simulink model "CurrentComp_LR_Vshunt_fb_v60"  (R2013a)
settings: Solver=ode23  StartTime=0.0  StopTime=1.2e-4  FixedStep=FS/50  MaxStep=1e-6  RelTol=1e-3  AbsTol=1e-5
InitFcn:
  | param=evalin('base','param;');
  | 
  | JR=str2num(param.JR);
  | KMT=str2num(param.KMT);
  | Rc=str2num(param.Rc);
  | Lc=str2num(param.Lc);
  | KFR=str2num(param.KFR);
  | KTB=str2num(param.KTB);
  | KBM=str2num(param.KBM);
  | Rsh=str2num(param.Rsh);
StartFcn:
  | sprintf('Info (%s):\nKTB = %.1e\nKBM = %.1e\n', gcs, KTB, KBM)
model workspace (MATLAB code in the model file):
  | %param=evalin('base','loadGalvoParam(4);');
  | param=evalin('base','param;');
  | 
  | JR=str2num(param.JR);
  | KMT=str2num(param.KMT);
  | Rc=str2num(param.Rc);
  | Lc=str2num(param.Lc);
  | KFR=str2num(param.KFR);
  | KTB=str2num(param.KTB);
  | KBM=str2num(param.KBM);
  | Rsh=str2num(param.Rsh);
libraries: simulink x1
settings Model: BufferReuse=off  Creator=mainster  LastModifiedBy=mainster
settings DataIOCC: SaveOutput=off  SaveTime=off
settings OptimizationCC: BlockReduction=off  InlineParams=on  OptimizeBlockIOStorage=off  BufferReuse=off  ExpressionFolding=off  LocalBlockOutputs=off
settings DebuggingCC: InitInArrayFormatMsg=none
settings ModelReferenceCC: ModelReferenceNumInstancesAllowed=Single  ModelReferenceMinAlgLoopOccurrences=on

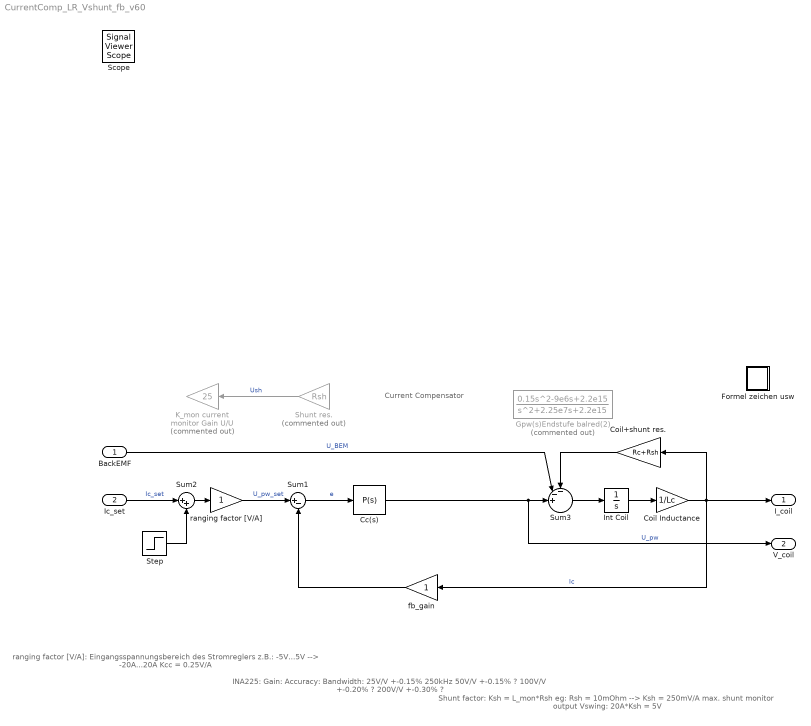
== system CurrentComp_LR_Vshunt_fb_v60 ==
  note: ranging factor [V/A]:
      | Eingangsspannungsbereich des
      | Stromreglers z.B.:
      | -5V...5V --> -20A...20A
      | Kcc = 0.25V/A
  note: Shunt factor:
      | Ksh = L_mon*Rsh
      |
      | eg: Rsh = 10mOhm
      |
      | --> Ksh = 250mV/A
      | max. shunt monitor
      | output Vswing:
      | 20A*Ksh = 5V
  note: INA225:
      | Gain:		Accuracy:		Bandwidth:
      | 25V/V		+-0.15%		250kHz
      | 50V/V		+-0.15%		?
      | 100V/V	+-0.20%		?
      | 200V/V	+-0.30%		?
  note: Current Compensator
  BackEMF : Inport
  Ic_set : Inport  Port=2
  Cc(s) : simulink/Continuous/PID Controller  Controller=P  TimeDomain=Continuous-time  SampleTime=-1  IntegratorMethod=Forward Euler  FilterMethod=Forward Euler  Form=Ideal  P=37.1538329650542  I=1985.39023021624  D=0  N=100  InitialConditionSource=internal  InitialConditionForIntegrator=0  InitialConditionForFilter=0  ExternalReset=none  LimitOutput=off  UpperSaturationLimit=inf  LowerSaturationLimit=-inf  LinearizeAsGain=on  AntiWindupMode=none  Kb=1  TrackingMode=off  Kt=1  PParamMin=[]  PParamMax=[]  IParamMin=[]  IParamMax=[]  DParamMin=[]  DParamMax=[]  NParamMin=[]  NParamMax=[]  KbParamMin=[]  KbParamMax=[]  KtParamMin=[]  KtParamMax=[]  POutMin=[]  POutMax=[]  IOutMin=[]  IOutMax=[]  DOutMin=[]  DOutMax=[]  NOutMin=[]  NOutMax=[]  KbOutMin=[]  KbOutMax=[]  KtOutMin=[]  KtOutMax=[]  IntegratorOutMin=[]  IntegratorOutMax=[]  FilterOutMin=[]  FilterOutMax=[]  SumOutMin=[]  SumOutMax=[]  SumI1OutMin=[]  SumI1OutMax=[]  SumI2OutMin=[]  SumI2OutMax=[]  SumI3OutMin=[]  SumI3OutMax=[]  SumDOutMin=[]  SumDOutMax=[]  SaturationOutMin=[]  SaturationOutMax=[]  IntegratorContinuousStateAttributes=''  IntegratorStateMustResolveToSignalObject=off  IntegratorRTWStateStorageClass=Auto  FilterContinuousStateAttributes=''  FilterStateMustResolveToSignalObject=off  FilterRTWStateStorageClass=Auto
      settings: AttributesFormatString=P = %<P>
  Coil Inductance : Gain  Gain=1/Lc
  Coil+shunt res. : Gain  Gain=Rc+Rsh
  Formel zeichen usw : Subsystem
  Gpw(s)Endstufe balred(2) : TransferFcn  Commented=on  Numerator=[0.15 -9e6 2.2e15]  Denominator=[1 2.25e7 2.2e15]
  Int Coil : Integrator
  K_mon current monitor Gain U/U : Gain  Commented=on  Gain=25
  Shunt res. : Gain  Commented=on  Gain=Rsh
  Step : Step  Time=0
      settings: AttributesFormatString=%<Time>
  Sum1 : Sum  Inputs=|+-
  Sum2 : Sum  Inputs=|++
  Sum3 : Sum  Inputs=--+||
  fb_gain : Gain
  ranging factor [V/A] : Gain
  I_coil : Outport
  V_coil : Outport  Port=2
  Scope : SignalViewerScope  IOType=viewer  RefreshTime=0.035000
      settings: ShowLegends=on  TimeRange=0.00014  YMin=-0.1  YMax=0.3
  wires:
  Ic_set/1 -> Sum2/1  "Ic_set"
  Sum1/1 -> Cc(s)/1  "e"
  Coil Inductance/1 -> fb_gain/1, I_coil/1, Coil+shunt res./1  "Ic"
  Sum3/1 -> Int Coil/1
  Int Coil/1 -> Coil Inductance/1
  Cc(s)/1 -> V_coil/1, Sum3/3  "U_pw"
  fb_gain/1 -> Sum1/2
  BackEMF/1 -> Sum3/2  "U_BEM"
  Coil+shunt res./1 -> Sum3/1
  ranging factor [V/A]/1 -> Sum1/1  "U_pw_set"
  Sum2/1 -> ranging factor [V/A]/1
  Step/1 -> Sum2/2
  Shunt res./1 -> K_mon current monitor Gain U/U/1  "Ush"

== system CurrentComp_LR_Vshunt_fb_v60/Formel zeichen usw ==
  note: Te: 		electrical torque, gen. by coils		[Nm]
      |  Ic: 			coil current							[A]
      |  Tfr:		rotor dynamic friction torque 		[Nm]
      |  Trb:		torsion bar torque					[Nm]
      |  Tw:		angular momentum				[Nm*s]
      |  w:			angular velocity 					[rad/s]
      |  yrad:		angular position 					[rad]
      |  ydeg:		angular position 					[°]
      |  Ucci:		current controller input				[V]
      |  Ucco:		current controller output			[V]
      |  Ush:		shunt voltage						[V]
  note: L_{c  }	coil inductance 							[H]
      |  R_{c  }	coil resistance							[\Omega]
      |  R_{SH }	current shunt resistance				[\Omega]
      |  J_{R  }	rotor inertia 							[kg*m²]
      |  K_{TB }	torsion bar torque const. 			[Nm/rad]
      |  K_{BM }	back EMF const.							[V*s/rad]
      |  K_{FR }	rotor dyn. friction torque const.	[Nm*s/rad]
      |  K_{MT }	el. magnetic torque const.			[Nm/A]
  note: balance of force: 	Te=Ttb+Tfr
      | 					Te - (Ttb+Tfr)=0  ->  no movement
      |
      |  integrate( 1 Nm )dt = 1 Nm*s
      |  (Nm*s)(kg*m²)⁻¹ = (N*s/kg)*m⁻¹ = m/(s*m) = rad
